simulink model "bldc_sixstep_f28069mLaunchPad"  (R2023b)
settings: Solver=FixedStepAuto  StartTime=0.0  StopTime=1.6  RelTol=1e-3  EnableMultiTasking=on
values from neighbouring files (symbols this model uses):
  bldc = mcb_SetPMSMMotorParameters('Teknic2310P')    [bldc_sixstep_f28069mLaunchPad_data.m]    (also in projectData.mat = )
  inverter = mcb_SetInverterParameters('BoostXL-DRV8305')    [bldc_sixstep_f28069mLaunchPad_data.m]    (also in projectData.mat = )
  PI_params = mcb_SetControllerParameters(bldc,inverter,PU_System,T_pwm,2*Ts,Ts_speed)    [bldc_sixstep_f28069mLaunchPad_data.m]    (also in projectData.mat = )
  PWM_frequency = 20e3    (= 20000)    [bldc_sixstep_f28069mLaunchPad_data.m]    (also in projectData.mat)
  target = mcb_SetProcessorDetails('F28069M',PWM_frequency)    [bldc_sixstep_f28069mLaunchPad_data.m]    (also in projectData.mat = )
  Ts = T_pwm    (= 5e-05)    [bldc_sixstep_f28069mLaunchPad_data.m]    (also in projectData.mat)
  Ts_motor_simscape = T_pwm/100    (= 5e-07)    [bldc_sixstep_f28069mLaunchPad_data.m]    (also in projectData.mat)
  Ts_simulink = T_pwm/2    (= 2.5e-05)    [bldc_sixstep_f28069mLaunchPad_data.m]    (also in projectData.mat)
  Ts_speed = 10*Ts    (= 0.0005)    [bldc_sixstep_f28069mLaunchPad_data.m]    (also in projectData.mat)
libraries: nesl_utility x14, fl_lib x9, mcbcontrolslib x7, simulink x6, pil_lib x6, ee_lib x5, slpidlib x4, mcbpositiondecoderlib x4
(part 1 of 3)
settings Model: ExtModeTrigDuration=8  Creator=Tefilus  LastModifiedBy=Tefilus
settings SolverCC: AutoInsertRateTranBlk=on
settings OptimizationCC: DefaultParameterBehavior=Inlined  DefaultUnderspecifiedDataType=single  EnhancedBackFolding=on  PassReuseOutputArgsAs=Individual arguments  MaxStackSize=1024  OptimizeBlockOrder=speed  DifferentSizesBufferReuse=on  OptimizationCustomize=off  DenormalBehavior=FlushToZero  EfficientTunableParamExpr=on
settings DebuggingCC: ParameterPrecisionLossMsg=none  ParameterTunabilityLossMsg=error
settings HardwareCC: ProdBitPerChar=16  ProdBitPerInt=16  ProdBitPerPointer=32  ProdBitPerSizeT=32  ProdBitPerPtrDiffT=32  ProdLargestAtomicInteger=Integer  ProdLargestAtomicFloat=None  ProdWordSize=16  ProdLongLongMode=on  ProdHWDeviceType=Texas Instruments->C2000  HardwareBoardFeatureSet=SoCBlockset
settings ModelReferenceCC: ModelReferenceNumInstancesAllowed=Single
settings SFSimCC: MATLABDynamicMemAlloc=off
settings RTWCC: Description=Embedded Coder  SystemTargetFile=ert.tlc  HardwareBoard=TI Piccolo F28069M LaunchPad  TemplateMakefile=ert_default_tmf  Toolchain=Texas Instruments Code Composer Studio (C2000)  PortableWordSizes=on  CreateSILPILBlock=PIL  CodeExecutionProfiling=on  CodeProfilingInstrumentation=coarse
settings CodeAppCC: ForceParamTrailComments=on  IgnoreCustomStorageClasses=off  OperatorAnnotations=on  SimulinkDataObjDesc=on  SFDataObjDesc=on  InsertBlockDesc=on
settings ERTTargetCC: CodeReplacementLibrary=TI C28x  ExtModeTransport=4  ExtModeStaticAlloc=on  ExtModeAutomaticAllocSize=off  ExtModeStaticAllocSize=2000  ExtModeMexFile=ext_xcp  ExtModeIntrfLevel=Level2 - Open  InlinedParameterPlacement=NonHierarchical

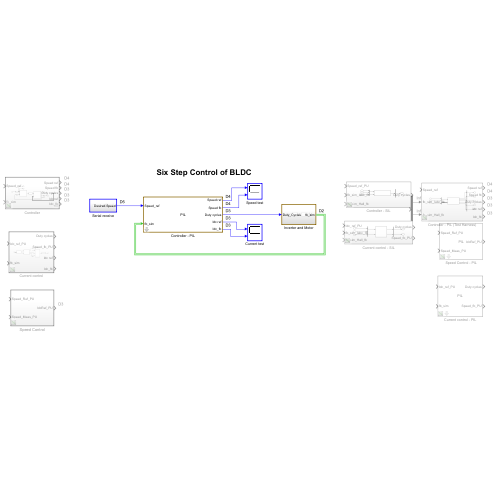
[thumbnail: Simulink's stored preview of the top-level diagram]
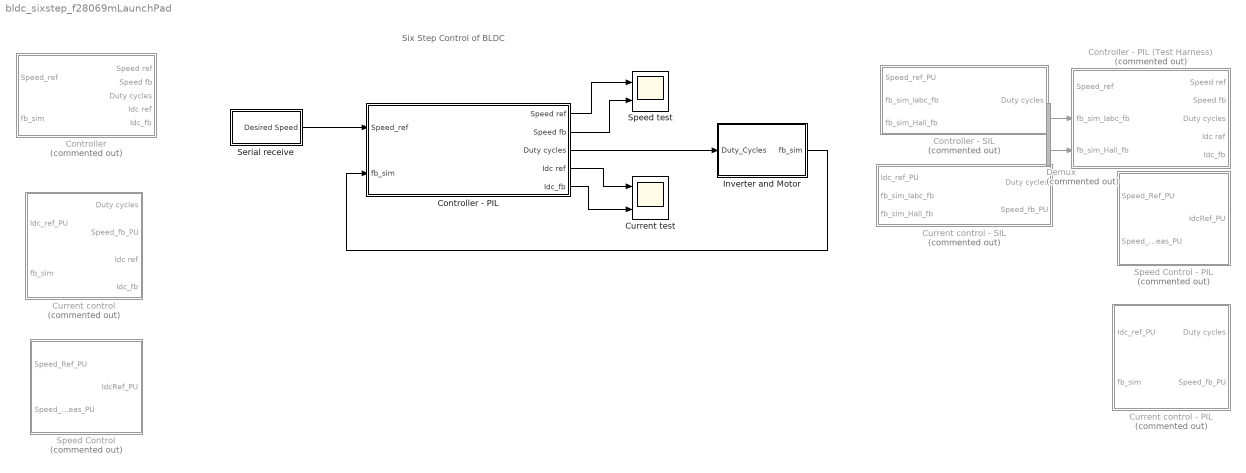
== system bldc_sixstep_f28069mLaunchPad ==
  note: Six Step Control of BLDC
  Controller : Subsystem  Commented=on  TreatAsAtomicUnit=on
  Controller - PIL : Subsystem  DialogController=pil_create_dialog  LoadFcn=|
      | try
      |    if ~strcmp(rtw.pil.getPILVersion, '23.2 (R2023b)_15')
      |       set_param(gcb, 'DialogController', '');
      |       set_param(gcb, 'DialogControllerArgs', '');
      |    end
      | catch e
      |       set_param(gcb, 'DialogController', '');
      |       set_param(gcb, 'DialogControllerArgs', '');
      | end
      mask help: PIL:pil:XILBlockMaskDesc
      mask Display: disp('PIL');
  Controller - PIL (Test Harness) : Subsystem  Commented=on
  Controller - SIL : Subsystem  Commented=on
  Current control : Subsystem  Commented=on  TreatAsAtomicUnit=on  SystemSampleTime=Ts
  Current control - PIL : Subsystem  Commented=on  DialogController=pil_create_dialog  LoadFcn=|
      | try
      |    if ~strcmp(rtw.pil.getPILVersion, '23.2 (R2023b)_15')
      |       set_param(gcb, 'DialogController', '');
      |       set_param(gcb, 'DialogControllerArgs', '');
      |    end
      | catch e
      |       set_param(gcb, 'DialogController', '');
      |       set_param(gcb, 'DialogControllerArgs', '');
      | end
      mask help: PIL:pil:XILBlockMaskDesc
      mask Display: disp('PIL');
  Current control - SIL : Subsystem  Commented=on
  Current test : Scope  NumInputPorts=2
  Demux : Demux  Commented=on  Outputs=2
  Inverter and Motor : Subsystem
  Serial receive : Subsystem  TreatAsAtomicUnit=on  SystemSampleTime=0.1
  Speed Control : Subsystem  Commented=on  TreatAsAtomicUnit=on  SystemSampleTime=Ts_speed
  Speed Control - PIL : Subsystem  Commented=on  DialogController=pil_create_dialog  LoadFcn=|
      | try
      |    if ~strcmp(rtw.pil.getPILVersion, '23.2 (R2023b)_15')
      |       set_param(gcb, 'DialogController', '');
      |       set_param(gcb, 'DialogControllerArgs', '');
      |    end
      | catch e
      |       set_param(gcb, 'DialogController', '');
      |       set_param(gcb, 'DialogControllerArgs', '');
      | end
      mask help: PIL:pil:XILBlockMaskDesc
      mask Display: disp('PIL');
  Speed test : Scope  NumInputPorts=2
  wires:
  Demux/1 -> Controller - PIL (Test Harness)/2(fb_sim_Iabc_fb)
  Demux/2 -> Controller - PIL (Test Harness)/3(fb_sim_Hall_fb)
  Controller - PIL/1(Speed ref) -> Speed test/1
  Controller - PIL/2(Speed fb) -> Speed test/2
  Controller - PIL/4(Idc ref) -> Current test/1
  Controller - PIL/5(Idc_fb) -> Current test/2
  Serial receive/1(Desired Speed) -> Controller - PIL/1(Speed_ref)
  Controller - PIL/3(Duty cycles) -> Inverter and Motor/1(Duty_Cycles)
  Inverter and Motor/1(fb_sim) -> Controller - PIL/2(fb_sim)

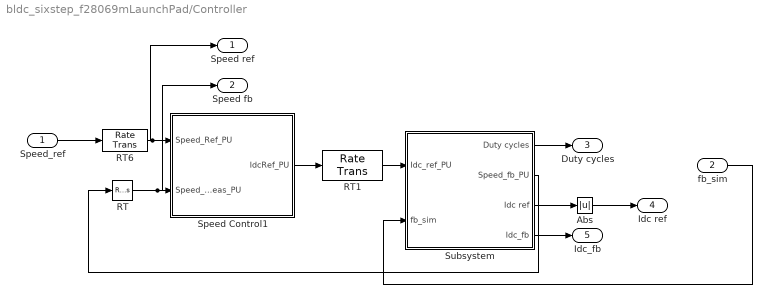
== system bldc_sixstep_f28069mLaunchPad/Controller ==
  Speed_ref : Inport
  fb_sim : Inport  Port=2
  Abs : Abs  SaturateOnIntegerOverflow=off
  RT : RateTransition  OutPortSampleTime=0.0005
  RT1 : RateTransition  Deterministic=off
  RT6 : RateTransition  Deterministic=off
  Speed Control1 : Subsystem  TreatAsAtomicUnit=on  SystemSampleTime=Ts_speed
  Subsystem : Subsystem  TreatAsAtomicUnit=on  SystemSampleTime=Ts
  Speed ref : Outport
  Speed fb : Outport  Port=2
  Duty cycles : Outport  Port=3
  Idc ref : Outport  Port=4
  Idc_fb : Outport  Port=5
  wires:
  Subsystem/2(Speed_fb_PU) -> RT/1
  RT6/1 -> Speed ref/1, Speed Control1/1(Speed_Ref_PU)
  Subsystem/1(Duty cycles) -> Duty cycles/1
  RT/1 -> Speed fb/1, Speed Control1/2(Speed_Meas_PU)
  Speed Control1/1(IdcRef_PU) -> RT1/1
  RT1/1 -> Subsystem/1(Idc_ref_PU)
  Speed_ref/1 -> RT6/1
  fb_sim/1 -> Subsystem/2(fb_sim)
  Subsystem/3(Idc ref) -> Abs/1
  Subsystem/4(Idc_fb) -> Idc_fb/1
  Abs/1 -> Idc ref/1

== system bldc_sixstep_f28069mLaunchPad/Controller - PIL ==
  Speed_ref : Inport
  fb_sim : Inport  Port=2
  Controller_sfcn : pil_lib/PIL Block  SimulationMode=PIL  IsTopModelPIL=off  CodeDir=Controller_ert_rtw  AnchorDir=E:\GiaotrinhDH\DATN\exampleSIL_PIL_MIL_HIL\SixStep_QEP  ConfigName=Texas Instruments C2000 Base  XrelIsTopModelCode=on  XrelIsReusable=off  XrelDWorkNames={}  XrelDWorkTypes={}  XrelModelArgVals={}  XrelOrderedParamNames={}
  __InputSSForSFun__ : Subsystem
  __OutputSSForSFun__ : Subsystem
  Speed ref : Outport
  Speed fb : Outport  Port=2
  Duty cycles : Outport  Port=3
  Idc ref : Outport  Port=4
  Idc_fb : Outport  Port=5
  wires:
  Speed_ref/1 -> __InputSSForSFun__/1(Speed_ref)
  fb_sim/1 -> __InputSSForSFun__/2(fb_sim)
  __InputSSForSFun__/1(__UniqueOutportName__1__) -> Controller_sfcn/1
  __InputSSForSFun__/2(__UniqueOutportName__2__) -> Controller_sfcn/2
  __InputSSForSFun__/3(__UniqueOutportName__3__) -> Controller_sfcn/3
  Controller_sfcn/1 -> __OutputSSForSFun__/1(__UniqueInportName__1__)
  Controller_sfcn/2 -> __OutputSSForSFun__/2(__UniqueInportName__2__)
  Controller_sfcn/3 -> __OutputSSForSFun__/3(__UniqueInportName__3__)
  Controller_sfcn/4 -> __OutputSSForSFun__/4(__UniqueInportName__4__)
  Controller_sfcn/5 -> __OutputSSForSFun__/5(__UniqueInportName__5__)
  __OutputSSForSFun__/1(Speed ref) -> Speed ref/1
  __OutputSSForSFun__/2(Speed fb) -> Speed fb/1
  __OutputSSForSFun__/3(Duty cycles) -> Duty cycles/1
  __OutputSSForSFun__/4(Idc ref) -> Idc ref/1
  __OutputSSForSFun__/5(Idc_fb) -> Idc_fb/1

== system bldc_sixstep_f28069mLaunchPad/Controller - PIL (Test Harness) ==
  Speed_ref : Inport  OutDataTypeStr=single  PortDimensions=[1]  SampleTime=0.1
  fb_sim_Iabc_fb : Inport  Port=2  OutDataTypeStr=uint16  PortDimensions=[3]  SampleTime=2.5e-05
  fb_sim_Hall_fb : Inport  Port=3  OutDataTypeStr=uint32  PortDimensions=[3]  SampleTime=5e-05
  Controller1 : Subsystem  Tag=__SL_testing_harness_stub_  DialogController=pil_create_dialog  LoadFcn=|
      | try
      |    if ~strcmp(rtw.pil.getPILVersion, '23.2 (R2023b)_15')
      |       set_param(gcb, 'DialogController', '');
      |       set_param(gcb, 'DialogControllerArgs', '');
      |    end
      | catch e
      |       set_param(gcb, 'DialogController', '');
      |       set_param(gcb, 'DialogControllerArgs', '');
      | end
      mask help: PIL:pil:XILBlockMaskDesc
      mask Display: disp('PIL');
  Input Conversion Subsystem : Subsystem  Tag=__SLT_ICS__  Description=|
      | Signal spec.
      | and routing
      settings: AttributesFormatString=%<Description>
  Output Conversion Subsystem : Subsystem  Tag=__SLT_OCS__  Description=|
      | Signal spec.
      | and routing
      settings: AttributesFormatString=%<Description>
  Speed ref : Outport
  Speed fb : Outport  Port=2
  Duty cycles : Outport  Port=3
  Idc ref : Outport  Port=4
  Idc_fb : Outport  Port=5
  wires:
  Controller1/2(Speed fb) -> Output Conversion Subsystem/2(Inport_2)
  Output Conversion Subsystem/2(Outport_2) -> Speed fb/1
  Output Conversion Subsystem/4(Outport_4) -> Idc ref/1
  Input Conversion Subsystem/1(Outport_1) -> Controller1/1(Speed_ref)
  Output Conversion Subsystem/3(Outport_3) -> Duty cycles/1
  Output Conversion Subsystem/5(Outport_5) -> Idc_fb/1
  fb_sim_Iabc_fb/1 -> Input Conversion Subsystem/2(Inport_2)
  Controller1/4(Idc ref) -> Output Conversion Subsystem/4(Inport_4)
  Controller1/3(Duty cycles) -> Output Conversion Subsystem/3(Inport_3)
  fb_sim_Hall_fb/1 -> Input Conversion Subsystem/3(Inport_3)
  Speed_ref/1 -> Input Conversion Subsystem/1(Inport_1)
  Output Conversion Subsystem/1(Outport_1) -> Speed ref/1
  Input Conversion Subsystem/2(Outport_2) -> Controller1/2(fb_sim)
  Controller1/1(Speed ref) -> Output Conversion Subsystem/1(Inport_1)
  Controller1/5(Idc_fb) -> Output Conversion Subsystem/5(Inport_5)

== system bldc_sixstep_f28069mLaunchPad/Controller - SIL ==
  Speed_ref_PU : Inport  OutDataTypeStr=single  PortDimensions=[1]  SampleTime=0.1
  fb_sim_Iabc_fb : Inport  Port=2  OutDataTypeStr=uint16  PortDimensions=[3]  SampleTime=2.5e-05
  fb_sim_Hall_fb : Inport  Port=3  OutDataTypeStr=uint32  PortDimensions=[3]  SampleTime=2.5e-05
  Input Conversion Subsystem : Subsystem  Tag=__SLT_ICS__  Description=|
      | Signal spec.
      | and routing
      settings: AttributesFormatString=%<Description>
  Output Conversion Subsystem : Subsystem  Tag=__SLT_OCS__  Description=|
      | Signal spec.
      | and routing
      settings: AttributesFormatString=%<Description>
  Subsystem : Subsystem  Tag=__SL_testing_harness_stub_  DialogController=pil_create_dialog  LoadFcn=|
      | try
      |    if ~strcmp(rtw.pil.getPILVersion, '23.2 (R2023b)_15')
      |       set_param(gcb, 'DialogController', '');
      |       set_param(gcb, 'DialogControllerArgs', '');
      |    end
      | catch e
      |       set_param(gcb, 'DialogController', '');
      |       set_param(gcb, 'DialogControllerArgs', '');
      | end
      mask help: PIL:pil:XILBlockMaskDesc
      mask Display: disp('SIL');
  Duty cycles : Outport
  wires:
  Speed_ref_PU/1 -> Input Conversion Subsystem/1(Inport_1)
  Input Conversion Subsystem/2(Outport_2) -> Subsystem/2(fb_sim)
  fb_sim_Hall_fb/1 -> Input Conversion Subsystem/3(Inport_3)
  fb_sim_Iabc_fb/1 -> Input Conversion Subsystem/2(Inport_2)
  Subsystem/1(Duty cycles) -> Output Conversion Subsystem/1(Inport_1)
  Output Conversion Subsystem/1(Outport_1) -> Duty cycles/1
  Input Conversion Subsystem/1(Outport_1) -> Subsystem/1(Speed_ref_PU)

== system bldc_sixstep_f28069mLaunchPad/Current control ==
  Idc_ref_PU : Inport
  fb_sim : Inport  Port=2
  Control_System : Subsystem
  Input scaling : Subsystem
  Inverter : Subsystem
  Sensor Driver Block : Subsystem
  Duty cycles : Outport
  Speed_fb_PU : Outport  Port=2
  Idc ref : Outport  Port=3
  Idc_fb : Outport  Port=4
  wires:
  fb_sim/1 -> Sensor Driver Block/1(fb_sim)
  Control_System/1(Duty) -> Inverter/1(Inverter Signals)
  Inverter/1(Duty) -> Duty cycles/1
  Idc_ref_PU/1 -> Idc ref/1, Control_System/1(Idc_ref_PU)
  Sensor Driver Block/1(Iabc_Meas_ADC) -> Input scaling/1(Iabc_meas_ADC)
  Sensor Driver Block/2(Hall_Meas) -> Input scaling/2(Hall_Meas)
  Input scaling/2(HallState) -> Control_System/2(Hallstate)
  Input scaling/3(Idc_meas_PU) -> Idc_fb/1, Control_System/3(Idc_fb_PU)
  Input scaling/1(speed_PU) -> Speed_fb_PU/1

== system bldc_sixstep_f28069mLaunchPad/Current control - PIL ==
  Idc_ref_PU : Inport
  fb_sim : Inport  Port=2
  Current control_sfcn : pil_lib/PIL Block  SimulationMode=PIL  IsTopModelPIL=off  CodeDir=Current_ert_rtw  AnchorDir=E:\GiaotrinhDH\DATN\exampleSIL_PIL_MIL_HIL\SixStep_QEP  ConfigName=Texas Instruments C2000 Base  XrelIsTopModelCode=on  XrelIsReusable=off  XrelDWorkNames={}  XrelDWorkTypes={}  XrelModelArgVals={}  XrelOrderedParamNames={}
  Scope : Scope  NumInputPorts=2
  __InputSSForSFun__ : Subsystem
  __OutputSSForSFun__ : Subsystem
  Duty cycles : Outport
  Speed_fb_PU : Outport  Port=2
  wires:
  Idc_ref_PU/1 -> __InputSSForSFun__/1(Idc_ref_PU)
  fb_sim/1 -> __InputSSForSFun__/2(fb_sim)
  __InputSSForSFun__/1(__UniqueOutportName__1__) -> Scope/1, Current control_sfcn/1
  __InputSSForSFun__/2(__UniqueOutportName__2__) -> Scope/2, Current control_sfcn/2
  __InputSSForSFun__/3(__UniqueOutportName__3__) -> Current control_sfcn/3
  Current control_sfcn/1 -> __OutputSSForSFun__/1(__UniqueInportName__1__)
  Current control_sfcn/2 -> __OutputSSForSFun__/2(__UniqueInportName__2__)
  __OutputSSForSFun__/1(Duty cycles) -> Duty cycles/1
  __OutputSSForSFun__/2(Speed_fb_PU) -> Speed_fb_PU/1

== system bldc_sixstep_f28069mLaunchPad/Current control - SIL ==
  Idc_ref_PU : Inport  OutDataTypeStr=single  PortDimensions=[1]  SampleTime=5e-05
  fb_sim_Iabc_fb : Inport  Port=2  OutDataTypeStr=uint16  PortDimensions=[3]  SampleTime=2.5e-05
  fb_sim_Hall_fb : Inport  Port=3  OutDataTypeStr=uint32  PortDimensions=[3]  SampleTime=2.5e-05
  Current control - SIL : Subsystem  Tag=__SL_testing_harness_stub_  DialogController=pil_create_dialog  LoadFcn=|
      | try
      |    if ~strcmp(rtw.pil.getPILVersion, '23.2 (R2023b)_15')
      |       set_param(gcb, 'DialogController', '');
      |       set_param(gcb, 'DialogControllerArgs', '');
      |    end
      | catch e
      |       set_param(gcb, 'DialogController', '');
      |       set_param(gcb, 'DialogControllerArgs', '');
      | end
      mask help: PIL:pil:XILBlockMaskDesc
      mask Display: disp('SIL');
  Input Conversion Subsystem : Subsystem  Tag=__SLT_ICS__  Description=|
      | Signal spec.
      | and routing
      settings: AttributesFormatString=%<Description>
  Output Conversion Subsystem : Subsystem  Tag=__SLT_OCS__  Description=|
      | Signal spec.
      | and routing
      settings: AttributesFormatString=%<Description>
  Duty cycles : Outport
  Speed_fb_PU : Outport  Port=2
  wires:
  Current control - SIL/1(Duty cycles) -> Output Conversion Subsystem/1(Inport_1)
  Output Conversion Subsystem/2(Outport_2) -> Speed_fb_PU/1
  Input Conversion Subsystem/2(Outport_2) -> Current control - SIL/2(fb_sim)
  fb_sim_Iabc_fb/1 -> Input Conversion Subsystem/2(Inport_2)
  Input Conversion Subsystem/1(Outport_1) -> Current control - SIL/1(Idc_ref_PU)
  Output Conversion Subsystem/1(Outport_1) -> Duty cycles/1
  fb_sim_Hall_fb/1 -> Input Conversion Subsystem/3(Inport_3)
  Current control - SIL/2(Speed_fb_PU) -> Output Conversion Subsystem/2(Inport_2)
  Idc_ref_PU/1 -> Input Conversion Subsystem/1(Inport_1)

== system bldc_sixstep_f28069mLaunchPad/Inverter and Motor ==
  Duty_Cycles : Inport
  Bus Creator : BusCreator  Inputs=2
  Inverter and Motor : Subsystem  VariantControl=get_param([bdroot '/Plant'],'Value')=='0'
  Load_Profile (Torque) : Subsystem
  RT2 : RateTransition  Deterministic=off  OutPortSampleTime=Ts_simulink
  RT3 : RateTransition  Deterministic=off  OutPortSampleTime=Ts_simulink
  Sensor_Measurements : Subsystem
  fb_sim : Outport
  wires:
  RT3/1 -> Sensor_Measurements/1(Iabc meas)
  Sensor_Measurements/2(HallState) -> Bus Creator/2  "Hall_fb"
  Inverter and Motor/2(Hall) -> RT2/1
  Sensor_Measurements/1(Iabc meas ADC) -> Bus Creator/1  "Iabc_fb"
  RT2/1 -> Sensor_Measurements/2(Hall)
  Load_Profile (Torque)/1(Load_Trq) -> Inverter and Motor/2(Load)
  Inverter and Motor/1(Iabc) -> RT3/1
  Duty_Cycles/1 -> Inverter and Motor/1(Duty_Cycles)
  Bus Creator/1 -> fb_sim/1

== system bldc_sixstep_f28069mLaunchPad/Serial receive ==
  Data Type Conversion1 : DataTypeConversion  OutDataTypeStr=dataType  RndMeth=Simplest  SaturateOnIntegerOverflow=off
  Data Type Conversion3 : DataTypeConversion  OutDataTypeStr=boolean  RndMeth=Simplest  SaturateOnIntegerOverflow=off
  Data conditioning : Subsystem
  Demux1 : Demux  Outputs=2
  SCI_Rx : Subsystem
  Terminator : Terminator
  Desired Speed : Outport  VectorParamsAs1DForOutWhenUnconnected=off
  wires:
  SCI_Rx/1(Data) -> Data conditioning/1(Rx_In)
  Demux1/1 -> Data Type Conversion1/1
  Demux1/2 -> Data Type Conversion3/1
  Data Type Conversion1/1 -> Desired Speed/1
  Data conditioning/1(Rx_Out) -> Demux1/1
  Data Type Conversion3/1 -> Terminator/1

== system bldc_sixstep_f28069mLaunchPad/Speed Control ==
  Speed_Ref_PU : Inport
  Speed_Meas_PU : Inport  Port=2
  PI_Controller_Speed : Subsystem
  Scope : Scope  NumInputPorts=2
  Speed_Ref_Selector : Subsystem
  IdcRef_PU : Outport  VectorParamsAs1DForOutWhenUnconnected=off
  wires:
  PI_Controller_Speed/1(Idc_ref) -> IdcRef_PU/1
  Speed_Meas_PU/1 -> Scope/2, PI_Controller_Speed/2(N_fb), Speed_Ref_Selector/2(Speed_Ref_Open)  "Speed_fb"
  Speed_Ref_PU/1 -> Scope/1, Speed_Ref_Selector/1(Speed_Ref_In)  "SpeedRef"
  Speed_Ref_Selector/1(Speed_Ref_PU) -> PI_Controller_Speed/1(N_ref)  "Speed_Ref"

== system bldc_sixstep_f28069mLaunchPad/Speed Control - PIL ==
  Speed_Ref_PU : Inport
  Speed_Meas_PU : Inport  Port=2
  Speed Control_sfcn : pil_lib/PIL Block  SimulationMode=PIL  IsTopModelPIL=off  CodeDir=Speed_ert_rtw  AnchorDir=E:\GiaotrinhDH\DATN\exampleSIL_PIL_MIL_HIL\SixStep_QEP  ConfigName=Texas Instruments C2000 Base  XrelIsTopModelCode=on  XrelIsReusable=off  XrelDWorkNames={}  XrelDWorkTypes={}  XrelModelArgVals={}  XrelOrderedParamNames={}
  __InputSSForSFun__ : Subsystem
  __OutputSSForSFun__ : Subsystem
  IdcRef_PU : Outport  VectorParamsAs1DForOutWhenUnconnected=off
  wires:
  Speed_Ref_PU/1 -> __InputSSForSFun__/1(Speed_Ref_PU)
  Speed_Meas_PU/1 -> __InputSSForSFun__/2(Speed_Meas_PU)
  __InputSSForSFun__/1(__UniqueOutportName__1__) -> Speed Control_sfcn/1
  __InputSSForSFun__/2(__UniqueOutportName__2__) -> Speed Control_sfcn/2
  Speed Control_sfcn/1 -> __OutputSSForSFun__/1(__UniqueInportName__1__)
  __OutputSSForSFun__/1(IdcRef_PU) -> IdcRef_PU/1

== system bldc_sixstep_f28069mLaunchPad/Controller/Speed Control1 ==
  Speed_Ref_PU : Inport
  Speed_Meas_PU : Inport  Port=2
  PI_Controller_Speed : Subsystem
  Scope : Scope  NumInputPorts=2
  Speed_Ref_Selector : Subsystem
  IdcRef_PU : Outport  VectorParamsAs1DForOutWhenUnconnected=off
  wires:
  PI_Controller_Speed/1(Idc_ref) -> IdcRef_PU/1
  Speed_Meas_PU/1 -> Scope/2, PI_Controller_Speed/2(N_fb), Speed_Ref_Selector/2(Speed_Ref_Open)  "Speed_fb"
  Speed_Ref_PU/1 -> Scope/1, Speed_Ref_Selector/1(Speed_Ref_In)  "SpeedRef"
  Speed_Ref_Selector/1(Speed_Ref_PU) -> PI_Controller_Speed/1(N_ref)  "Speed_Ref"

== system bldc_sixstep_f28069mLaunchPad/Controller/Subsystem ==
  Idc_ref_PU : Inport
  fb_sim : Inport  Port=2
  Control_System : Subsystem
  Input scaling : Subsystem
  Inverter : Subsystem
  Sensor Driver Block : Subsystem
  Duty cycles : Outport
  Speed_fb_PU : Outport  Port=2
  Idc ref : Outport  Port=3
  Idc_fb : Outport  Port=4
  wires:
  fb_sim/1 -> Sensor Driver Block/1(fb_sim)
  Control_System/1(Duty) -> Inverter/1(Inverter Signals)
  Inverter/1(Duty) -> Duty cycles/1
  Idc_ref_PU/1 -> Idc ref/1, Control_System/1(Idc_ref_PU)
  Sensor Driver Block/1(Iabc_Meas_ADC) -> Input scaling/1(Iabc_meas_ADC)
  Sensor Driver Block/2(Hall_Meas) -> Input scaling/2(Hall_Meas)
  Input scaling/2(HallState) -> Control_System/2(Hallstate)
  Input scaling/3(Idc_meas_PU) -> Idc_fb/1, Control_System/3(Idc_fb_PU)
  Input scaling/1(speed_PU) -> Speed_fb_PU/1

== system bldc_sixstep_f28069mLaunchPad/Controller - PIL/__InputSSForSFun__ ==
  Speed_ref : Inport
  fb_sim : Inport  Port=2
  temporaryBusSelectName_1 : BusSelector  OutputSignals=Iabc_fb,Hall_fb
  __UniqueOutportName__1__ : Outport
  __UniqueOutportName__2__ : Outport  Port=2
  __UniqueOutportName__3__ : Outport  Port=3
  wires:
  fb_sim/1 -> temporaryBusSelectName_1/1
  Speed_ref/1 -> __UniqueOutportName__1__/1
  temporaryBusSelectName_1/1 -> __UniqueOutportName__2__/1  "<Iabc_fb>"
  temporaryBusSelectName_1/2 -> __UniqueOutportName__3__/1  "<Hall_fb>"

== system bldc_sixstep_f28069mLaunchPad/Controller - PIL/__OutputSSForSFun__ ==
  __UniqueInportName__1__ : Inport
  __UniqueInportName__2__ : Inport  Port=2
  __UniqueInportName__3__ : Inport  Port=3
  __UniqueInportName__4__ : Inport  Port=4
  __UniqueInportName__5__ : Inport  Port=5
  Speed ref : Outport
  Speed fb : Outport  Port=2
  Duty cycles : Outport  Port=3
  Idc ref : Outport  Port=4
  Idc_fb : Outport  Port=5
  wires:
  __UniqueInportName__1__/1 -> Speed ref/1
  __UniqueInportName__2__/1 -> Speed fb/1
  __UniqueInportName__3__/1 -> Duty cycles/1
  __UniqueInportName__4__/1 -> Idc ref/1
  __UniqueInportName__5__/1 -> Idc_fb/1  "IDC"

== system bldc_sixstep_f28069mLaunchPad/Controller - PIL (Test Harness)/Controller1 ==
  Speed_ref : Inport
  fb_sim : Inport  Port=2
  Controller_sfcn : pil_lib/PIL Block  SimulationMode=PIL  IsTopModelPIL=off  CodeDir=Controller_ert_rtw  AnchorDir=E:\GiaotrinhDH\DATN\exampleSIL_PIL_MIL_HIL\SixStep_QEP  ConfigName=Texas Instruments C2000 Base  XrelIsTopModelCode=on  XrelIsReusable=off  XrelDWorkNames={}  XrelDWorkTypes={}  XrelModelArgVals={}  XrelOrderedParamNames={}
  __InputSSForSFun__ : Subsystem
  __OutputSSForSFun__ : Subsystem
  Speed ref : Outport
  Speed fb : Outport  Port=2
  Duty cycles : Outport  Port=3
  Idc ref : Outport  Port=4
  Idc_fb : Outport  Port=5
  wires:
  __OutputSSForSFun__/5(Idc_fb) -> Idc_fb/1
  __OutputSSForSFun__/4(Idc ref) -> Idc ref/1
  __OutputSSForSFun__/3(Duty cycles) -> Duty cycles/1
  __OutputSSForSFun__/2(Speed fb) -> Speed fb/1
  __OutputSSForSFun__/1(Speed ref) -> Speed ref/1
  Controller_sfcn/5 -> __OutputSSForSFun__/5(__UniqueInportName__5__)
  Controller_sfcn/4 -> __OutputSSForSFun__/4(__UniqueInportName__4__)
  Controller_sfcn/3 -> __OutputSSForSFun__/3(__UniqueInportName__3__)
  Controller_sfcn/2 -> __OutputSSForSFun__/2(__UniqueInportName__2__)
  Controller_sfcn/1 -> __OutputSSForSFun__/1(__UniqueInportName__1__)
  __InputSSForSFun__/3(__UniqueOutportName__3__) -> Controller_sfcn/3
  __InputSSForSFun__/2(__UniqueOutportName__2__) -> Controller_sfcn/2
  __InputSSForSFun__/1(__UniqueOutportName__1__) -> Controller_sfcn/1
  fb_sim/1 -> __InputSSForSFun__/2(fb_sim)
  Speed_ref/1 -> __InputSSForSFun__/1(Speed_ref)

== system bldc_sixstep_f28069mLaunchPad/Controller - PIL (Test Harness)/Input Conversion Subsystem ==
  note: This subsystem has been inserted by Simulink to adapt the output of the source blocks to the interface required by the harnessed component.
      |  Modifying the contents of this subsystem may result in compilation and simulation failure.
  Inport_1 : Inport
  Inport_2 : Inport  Port=2
  Inport_3 : Inport  Port=3
  BusCreator_1 : BusCreator  Inputs=2
  SigSpec_1 : SignalSpecification  OutDataTypeStr=single  Dimensions=[1]  SampleTime=0.1
  SigSpec_2 : SignalSpecification  OutDataTypeStr=uint16  Dimensions=[3]  SampleTime=2.5e-05
  SigSpec_3 : SignalSpecification  OutDataTypeStr=uint32  Dimensions=[3]  SampleTime=5e-05
  Outport_1 : Outport
  Outport_2 : Outport  Port=2
  wires:
  SigSpec_1/1 -> Outport_1/1
  Inport_1/1 -> SigSpec_1/1
  BusCreator_1/1 -> Outport_2/1
  SigSpec_2/1 -> BusCreator_1/1
  Inport_2/1 -> SigSpec_2/1  "Iabc_fb"
  SigSpec_3/1 -> BusCreator_1/2
  Inport_3/1 -> SigSpec_3/1  "Hall_fb"

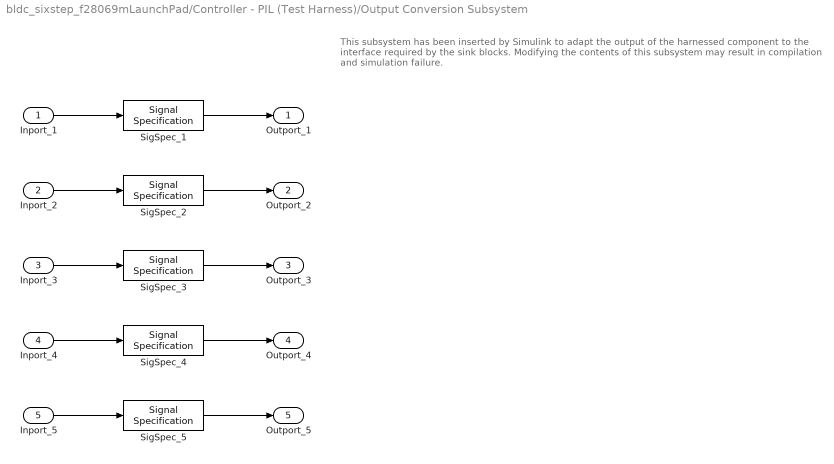
== system bldc_sixstep_f28069mLaunchPad/Controller - PIL (Test Harness)/Output Conversion Subsystem ==
  note: This subsystem has been inserted by Simulink to adapt the output of the harnessed component to the interface required by the sink blocks.
      |  Modifying the contents of this subsystem may result in compilation and simulation failure.
  Inport_1 : Inport
  Inport_2 : Inport  Port=2
  Inport_3 : Inport  Port=3
  Inport_4 : Inport  Port=4
  Inport_5 : Inport  Port=5
  SigSpec_1 : SignalSpecification  OutDataTypeStr=single  Dimensions=[1]  SampleTime=0.0005
  SigSpec_2 : SignalSpecification  OutDataTypeStr=single  Dimensions=[1]  SampleTime=0.0005
  SigSpec_3 : SignalSpecification  OutDataTypeStr=single  Dimensions=[6]  SampleTime=5e-05
  SigSpec_4 : SignalSpecification  OutDataTypeStr=single  Dimensions=[1]  SampleTime=5e-05
  SigSpec_5 : SignalSpecification  OutDataTypeStr=single  Dimensions=[1]  SampleTime=5e-05
  Outport_1 : Outport
  Outport_2 : Outport  Port=2
  Outport_3 : Outport  Port=3
  Outport_4 : Outport  Port=4
  Outport_5 : Outport  Port=5
  wires:
  Inport_1/1 -> SigSpec_1/1
  SigSpec_1/1 -> Outport_1/1
  Inport_2/1 -> SigSpec_2/1
  SigSpec_2/1 -> Outport_2/1
  Inport_3/1 -> SigSpec_3/1
  SigSpec_3/1 -> Outport_3/1
  Inport_4/1 -> SigSpec_4/1
  SigSpec_4/1 -> Outport_4/1
  Inport_5/1 -> SigSpec_5/1
  SigSpec_5/1 -> Outport_5/1

== system bldc_sixstep_f28069mLaunchPad/Controller - SIL/Input Conversion Subsystem ==
  note: This subsystem has been inserted by Simulink to adapt the output of the source blocks to the interface required by the harnessed component.
      |  Modifying the contents of this subsystem may result in compilation and simulation failure.
  Inport_1 : Inport
  Inport_2 : Inport  Port=2
  Inport_3 : Inport  Port=3
  BusCreator_1 : BusCreator  Inputs=2
  SigSpec_1 : SignalSpecification  OutDataTypeStr=single  Dimensions=[1]  SampleTime=0.1
  SigSpec_2 : SignalSpecification  OutDataTypeStr=uint16  Dimensions=[3]  SampleTime=2.5e-05
  SigSpec_3 : SignalSpecification  OutDataTypeStr=uint32  Dimensions=[3]  SampleTime=2.5e-05
  Outport_1 : Outport
  Outport_2 : Outport  Port=2
  wires:
  SigSpec_1/1 -> Outport_1/1
  Inport_1/1 -> SigSpec_1/1
  BusCreator_1/1 -> Outport_2/1
  SigSpec_2/1 -> BusCreator_1/1
  Inport_2/1 -> SigSpec_2/1  "Iabc_fb"
  SigSpec_3/1 -> BusCreator_1/2
  Inport_3/1 -> SigSpec_3/1  "Hall_fb"

== system bldc_sixstep_f28069mLaunchPad/Controller - SIL/Output Conversion Subsystem ==
  note: This subsystem has been inserted by Simulink to adapt the output of the harnessed component to the interface required by the sink blocks.
      |  Modifying the contents of this subsystem may result in compilation and simulation failure.
  Inport_1 : Inport
  SigSpec_1 : SignalSpecification  OutDataTypeStr=single  Dimensions=[6]  SampleTime=5e-05
  Outport_1 : Outport
  wires:
  Inport_1/1 -> SigSpec_1/1
  SigSpec_1/1 -> Outport_1/1

== system bldc_sixstep_f28069mLaunchPad/Controller - SIL/Subsystem ==
  Speed_ref_PU : Inport
  fb_sim : Inport  Port=2
  Subsystem_sfcn : pil_lib/PIL Block  SimulationMode=SIL  IsTopModelPIL=off  CodeDir=Subsystem_ert_rtw  AnchorDir=E:\GiaotrinhDH\DATN\exampleSIL_PIL_MIL_HIL\SixStep_QEP  ConfigName=Software-in-the-Loop (SIL)  XrelIsTopModelCode=on  XrelIsReusable=off  XrelDWorkNames={}  XrelDWorkTypes={}  XrelModelArgVals={}  XrelOrderedParamNames={}
  __InputSSForSFun__ : Subsystem
  __OutputSSForSFun__ : Subsystem
  Duty cycles : Outport
  wires:
  __OutputSSForSFun__/1(Duty cycles) -> Duty cycles/1
  Subsystem_sfcn/1 -> __OutputSSForSFun__/1(__UniqueInportName__1__)
  __InputSSForSFun__/3(__UniqueOutportName__3__) -> Subsystem_sfcn/3
  __InputSSForSFun__/2(__UniqueOutportName__2__) -> Subsystem_sfcn/2
  __InputSSForSFun__/1(__UniqueOutportName__1__) -> Subsystem_sfcn/1
  fb_sim/1 -> __InputSSForSFun__/2(fb_sim)
  Speed_ref_PU/1 -> __InputSSForSFun__/1(Speed_ref_PU)

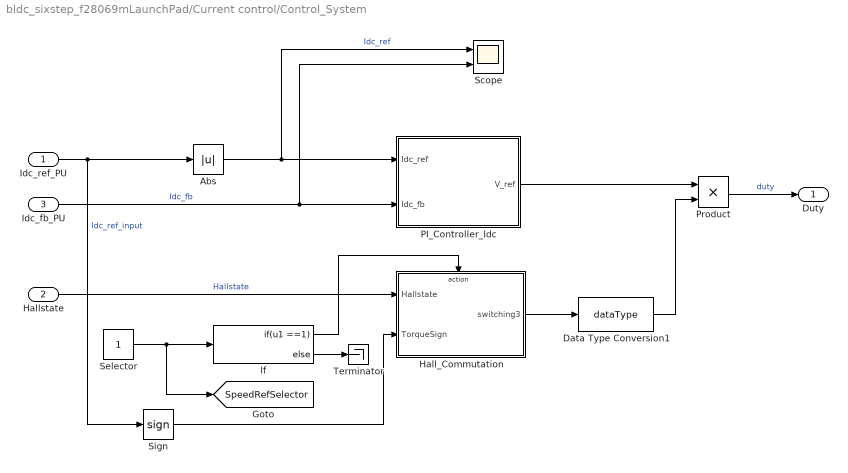
== system bldc_sixstep_f28069mLaunchPad/Current control/Control_System ==
  Idc_ref_PU : Inport
  Hallstate : Inport  Port=2
  Idc_fb_PU : Inport  Port=3
  Abs : Abs  SaturateOnIntegerOverflow=off
  Data Type Conversion1 : DataTypeConversion  OutDataTypeStr=dataType  RndMeth=Simplest  SaturateOnIntegerOverflow=off
  Hall_Commutation : Subsystem
  If : If  IfExpression=u1 ==1
  PI_Controller_Idc : Subsystem
  Product : Product  RndMeth=Simplest  OutDataTypeStr=Inherit: Same as first input
  Scope : Scope  NumInputPorts=2
  Selector : Constant  OutDataTypeStr=uint16  SampleTime=-1
  Sign : Signum
  Terminator : Terminator
  Duty : Outport  VectorParamsAs1DForOutWhenUnconnected=off
  tag scope: SpeedRefSelector=global
  wires:
  Hallstate/1 -> Hall_Commutation/1(Hallstate)  "Hallstate"
  If/1 -> Hall_Commutation/Action
  Idc_fb_PU/1 -> Scope/2, PI_Controller_Idc/2(Idc_fb)  "Idc_fb"
  Abs/1 -> Scope/1, PI_Controller_Idc/1(Idc_ref)  "Idc_ref"
  PI_Controller_Idc/1(V_ref) -> Product/1
  Idc_ref_PU/1 -> Sign/1, Abs/1  "Idc_ref_input"
  Product/1 -> Duty/1  "duty"
  Selector/1 -> If/1, [SpeedRefSelector]
  Sign/1 -> Hall_Commutation/2(TorqueSign)
  Data Type Conversion1/1 -> Product/2
  Hall_Commutation/1(switching3) -> Data Type Conversion1/1
  If/2 -> Terminator/1

== system bldc_sixstep_f28069mLaunchPad/Current control/Input scaling ==
  Iabc_meas_ADC : Inport
  Hall_Meas : Inport  Port=2
  Convert ADC value to PU : Subsystem
  Hall Feedback : Subsystem  TreatAsAtomicUnit=on
  Hall selected : Constant
  If : If  IfExpression=u1 ==1
  Terminator : Terminator
  Terminator1 : Terminator
  speed_PU : Outport  InitialOutput=0  VectorParamsAs1DForOutWhenUnconnected=off
  HallState : Outport  Port=2  InitialOutput=0  VectorParamsAs1DForOutWhenUnconnected=off
  Idc_meas_PU : Outport  Port=3
  wires:
  Hall Feedback/1(HallState) -> HallState/1
  Hall_Meas/1 -> Hall Feedback/1(Hall_Meas)
  If/1 -> Hall Feedback/Action
  Hall selected/1 -> If/1
  Hall Feedback/2(Speed_PU) -> speed_PU/1
  If/2 -> Terminator/1
  Iabc_meas_ADC/1 -> Convert ADC value to PU/1(Iabc_meas_ADC)
  Convert ADC value to PU/1(Idc_meas_PU) -> Idc_meas_PU/1
  Convert ADC value to PU/2(Ia_meas_PU) -> Terminator1/1

== system bldc_sixstep_f28069mLaunchPad/Current control/Inverter ==
  Inverter Signals : Inport
  Constant : Constant
  Data Type Duplicate : DataTypeDuplicate
  Switch : Switch  Threshold=0.5  RndMeth=Simplest  SaturateOnIntegerOverflow=off  InputSameDT=off
  stop : Constant  Value=[0 0 0 0 0 0]  OutDataTypeStr=Inherit: Inherit via back propagation
  Duty : Outport  VectorParamsAs1DForOutWhenUnconnected=off
  wires:
  Constant/1 -> Switch/2
  Switch/1 -> Duty/1
  Inverter Signals/1 -> Switch/1, Data Type Duplicate/1  "PWM Duty Cycles"
  stop/1 -> Switch/3, Data Type Duplicate/2

== system bldc_sixstep_f28069mLaunchPad/Current control/Sensor Driver Block ==
  fb_sim : Inport
  Bus Selector : BusSelector  OutputSignals=Iabc_fb,Hall_fb
  Iabc_Meas_ADC : Outport
  Hall_Meas : Outport  Port=2
  wires:
  Bus Selector/1 -> Iabc_Meas_ADC/1  "<Iabc_fb>"
  fb_sim/1 -> Bus Selector/1
  Bus Selector/2 -> Hall_Meas/1  "<Hall_fb>"

== system bldc_sixstep_f28069mLaunchPad/Current control - PIL/__InputSSForSFun__ ==
  Idc_ref_PU : Inport
  fb_sim : Inport  Port=2
  temporaryBusSelectName_1 : BusSelector  OutputSignals=Iabc_fb,Hall_fb
  __UniqueOutportName__1__ : Outport
  __UniqueOutportName__2__ : Outport  Port=2
  __UniqueOutportName__3__ : Outport  Port=3
  wires:
  fb_sim/1 -> temporaryBusSelectName_1/1
  Idc_ref_PU/1 -> __UniqueOutportName__1__/1
  temporaryBusSelectName_1/1 -> __UniqueOutportName__2__/1  "<Iabc_fb>"
  temporaryBusSelectName_1/2 -> __UniqueOutportName__3__/1  "<Hall_fb>"

== system bldc_sixstep_f28069mLaunchPad/Current control - PIL/__OutputSSForSFun__ ==
  __UniqueInportName__1__ : Inport
  __UniqueInportName__2__ : Inport  Port=2
  Duty cycles : Outport
  Speed_fb_PU : Outport  Port=2
  wires:
  __UniqueInportName__1__/1 -> Duty cycles/1
  __UniqueInportName__2__/1 -> Speed_fb_PU/1

== system bldc_sixstep_f28069mLaunchPad/Current control - SIL/Current control - SIL ==
  Idc_ref_PU : Inport
  fb_sim : Inport  Port=2
  Current control_sfcn : pil_lib/PIL Block  SimulationMode=SIL  IsTopModelPIL=off  CodeDir=Current_ert_rtw  AnchorDir=E:\GiaotrinhDH\DATN\exampleSIL_PIL_MIL_HIL\SixStep_QEP  ConfigName=Software-in-the-Loop (SIL)  XrelIsTopModelCode=on  XrelIsReusable=off  XrelDWorkNames={}  XrelDWorkTypes={}  XrelModelArgVals={}  XrelOrderedParamNames={}
  __InputSSForSFun__ : Subsystem
  __OutputSSForSFun__ : Subsystem
  Duty cycles : Outport
  Speed_fb_PU : Outport  Port=2
  wires:
  __OutputSSForSFun__/2(Speed_fb_PU) -> Speed_fb_PU/1
  __OutputSSForSFun__/1(Duty cycles) -> Duty cycles/1
  Current control_sfcn/2 -> __OutputSSForSFun__/2(__UniqueInportName__2__)
  Current control_sfcn/1 -> __OutputSSForSFun__/1(__UniqueInportName__1__)
  __InputSSForSFun__/3(__UniqueOutportName__3__) -> Current control_sfcn/3
  __InputSSForSFun__/2(__UniqueOutportName__2__) -> Current control_sfcn/2
  __InputSSForSFun__/1(__UniqueOutportName__1__) -> Current control_sfcn/1
  fb_sim/1 -> __InputSSForSFun__/2(fb_sim)
  Idc_ref_PU/1 -> __InputSSForSFun__/1(Idc_ref_PU)

== system bldc_sixstep_f28069mLaunchPad/Current control - SIL/Input Conversion Subsystem ==
  note: This subsystem has been inserted by Simulink to adapt the output of the source blocks to the interface required by the harnessed component.
      |  Modifying the contents of this subsystem may result in compilation and simulation failure.
  Inport_1 : Inport
  Inport_2 : Inport  Port=2
  Inport_3 : Inport  Port=3
  BusCreator_1 : BusCreator  Inputs=2
  SigSpec_1 : SignalSpecification  OutDataTypeStr=single  Dimensions=[1]  SampleTime=5e-05
  SigSpec_2 : SignalSpecification  OutDataTypeStr=uint16  Dimensions=[3]  SampleTime=2.5e-05
  SigSpec_3 : SignalSpecification  OutDataTypeStr=uint32  Dimensions=[3]  SampleTime=2.5e-05
  Outport_1 : Outport
  Outport_2 : Outport  Port=2
  wires:
  SigSpec_1/1 -> Outport_1/1
  Inport_1/1 -> SigSpec_1/1
  BusCreator_1/1 -> Outport_2/1
  SigSpec_2/1 -> BusCreator_1/1
  Inport_2/1 -> SigSpec_2/1  "Iabc_fb"
  SigSpec_3/1 -> BusCreator_1/2
  Inport_3/1 -> SigSpec_3/1  "Hall_fb"

== system bldc_sixstep_f28069mLaunchPad/Current control - SIL/Output Conversion Subsystem ==
  note: This subsystem has been inserted by Simulink to adapt the output of the harnessed component to the interface required by the sink blocks.
      |  Modifying the contents of this subsystem may result in compilation and simulation failure.
  Inport_1 : Inport
  Inport_2 : Inport  Port=2
  SigSpec_1 : SignalSpecification  OutDataTypeStr=single  Dimensions=[6]  SampleTime=5e-05
  SigSpec_2 : SignalSpecification  OutDataTypeStr=single  Dimensions=[1]  SampleTime=5e-05
  Outport_1 : Outport
  Outport_2 : Outport  Port=2
  wires:
  Inport_1/1 -> SigSpec_1/1
  SigSpec_1/1 -> Outport_1/1
  Inport_2/1 -> SigSpec_2/1
  SigSpec_2/1 -> Outport_2/1

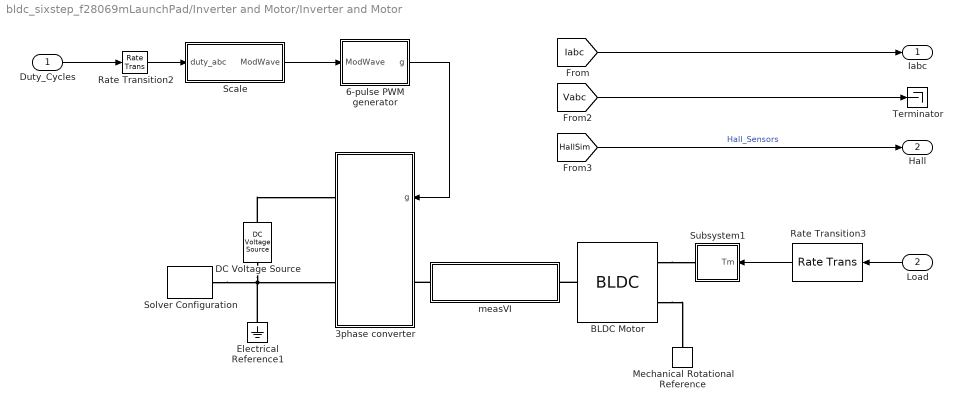
== system bldc_sixstep_f28069mLaunchPad/Inverter and Motor/Inverter and Motor ==
  Duty_Cycles : Inport
  Load : Inport  Port=2
  3phase converter : Subsystem
  6-pulse PWM generator : Subsystem  mask{fs=PWM_frequency}
      mask prompts: fs "Carrier Frequency (Hz)"
  BLDC Motor : ee_lib/Electromechanical/Permanent Magnet/BLDC  port_option=ee.enum.threePhasePort.composite  rotor_param=1  pm_flux_linkage=bldc.FluxPM Wb  theta_constant=pi /(2*bldc.p) rad  emf_max=9.6 V  w_meas=600 rpm  DphiDtheta_tab=[0, -.1528, -.1528, .1528, .1528, 0] Wb/rad  back_emf_tab=[0, -9.6, -9.6, 9.6, 9.6, 0] V  rotor_angle_tab=[0, 7.5, 22.5, 37.5, 52.5, 60] deg  nPolePairs=bldc.p  axes_param=2  winding_type=ee.enum.statorconnection.wye  stator_param=ee.enum.statorparam.LdLqL0  machine_param=ee.enum.dqparameterization.constant  Ld=bldc.Ld H  Lq=bldc.Lq H  idVec=[-200, 0, 200] A  iqVec=[-200, 0, 200] A  LdMatrix=0.00022 * ones(3, 3) H  LqMatrix=0.00022 * ones(3, 3) H  L0=0.00016 H  Ls=0.0002 H  Lm=0 H  Ms=0.00002 H  Rs=bldc.Rs Ohm  zero_sequence=ee.enum.park.zerosequence.exclude  loss_param=ee.enum.ironloss.none  losses_oc=[0, 0, 0] W  losses_sc=[0, 0, 0] W  f_losses=60 Hz  Isc_losses=95 A  J=bldc.J kg*m^2  lam=bldc.B N*m/(rad/s)  i_d_specify=off  i_d_priority=None  i_d=0 A  i_d_nominal_specify=off  i_d_nominal_unit=A  i_d_nominal_value=1  i_q_specify=off  i_q_priority=None  i_q=0 A  i_q_nominal_specify=off  i_q_nominal_unit=A  i_q_nominal_value=1  torque_specify=off  torque_priority=None  torque=0 N*m  torque_nominal_specify=off  torque_nominal_unit=N*m  torque_nominal_value=1  angular_velocity_specify=off  angular_velocity_priority=High  angular_velocity=0 rpm  angular_velocity_nominal_specify=off  angular_velocity_nominal_unit=rpm  angular_velocity_nominal_value=1  angular_position_specify=off  angular_position_priority=High  angular_position=0 deg  angular_position_nominal_specify=off  angular_position_nominal_unit=deg  angular_position_nominal_value=1  alpha=3.93e-3 1/K  alpha_flux=-0.001 1/K  Tmeas=298.15 K  stator_thermal_mass=100 J/K  rotor_thermal_mass=200 J/K  Rm_percent_rotor=90  Rd_percent_rotor=30  temperatureA_specify=off  temperatureA_priority=High  temperatureA=25 degC  temperatureA_nominal_specify=off  temperatureA_nominal_unit=degC  temperatureA_nominal_value=1  temperatureB_specify=off  temperatureB_priority=High  temperatureB=25 degC  temperatureB_nominal_specify=off  temperatureB_nominal_unit=degC  temperatureB_nominal_value=1  temperatureC_specify=off  temperatureC_priority=High  temperatureC=25 degC  temperatureC_nominal_specify=off  temperatureC_nominal_unit=degC  temperatureC_nominal_value=1  temperatureR_specify=off  temperatureR_priority=High  temperatureR=25 degC  temperatureR_nominal_specify=off  temperatureR_nominal_unit=degC  temperatureR_nominal_value=1
      settings: InternalSimscapePortConfiguration="{\"Bottom\":[],\"Left\":[{\"id\":\"N\",\"label\":\"~\",\"type\":\"foundation.electrical.three_phase\"}],\"Right\":[{\"id\":\"R\",\"label\":\"R\",\"type\":\"foundation.mechanical.rotational.rotational\"},{\"id\":\"C\",\"label\":\"C\",\"type\":\"foundation.mechanical.rotational.rotational\"}],\"Top\":[]}"
  DC Voltage Source : fl_lib/Electrical/Electrical Sources/DC Voltage Source  v0=inverter.V_dc V
  Electrical Reference1 : fl_lib/Electrical/Electrical Elements/Electrical Reference
  Mechanical Rotational Reference : fl_lib/Mechanical/Rotational Elements/Mechanical Rotational Reference
  Rate Transition2 : RateTransition  Deterministic=off  OutPortSampleTime=Ts_motor_simscape
  Rate Transition3 : RateTransition  Deterministic=off  OutPortSampleTime=Ts_motor_simscape
  Scale : Subsystem
  Solver Configuration : nesl_utility/Solver Configuration  PhysicalDomain=network_engine_domain  SubClassName=solver  LeftPortType=input  RightPortType=generic  Tones=[]  Harmonics=[]  SimulateNoise=off  Profile=off  UseLocalSampling=off  EnableSwitchedLinearOptims=on  FrequencyDomain=off  UseCCode=off  RelTol=0.001  AbsTol=1e-06  MinStep=1e-09  ToWorkspace=off  RevertToSquareIcSolve=off  NumHomotopyIterations=100  PhasorMode=off  PhasorModeNumHarmonics=1  ConsistencySolver=NEWTON_FTOL  IndexReductionMethod=DerivativeReplacement  DoDC=off  ResidualTolerance=1e-09  ConsistencyTolSource=GLOBAL  ConsistencyAbsTol=0.001  ConsistencyRelTol=0.001  ConsistencyTolFactor=0.001  UseLocalSolver=on  LocalSolverChoice=NE_PARTITIONING_ADVANCER  ResolveIndetEquations=on  FunctionEvalNumThread=1  LocalSolverSampleTime=Ts_motor_simscape  DoFixedCost=on  MaxNonlinIter=4  MaxModeIter=2  ComputeImpulses=off  ImpulseIterations=1  LinearAlgebra=auto  LinearAlgebraNumThread=0  EquationFormulation=NE_TIME_EF  DelaysMemoryBudget=1024  AutomaticFiltering=on  FilteringTimeConstant=0.001  PartitionStorageMethod=AS_NEEDED  PartitionMemoryBudget=1024  PartitionMethod=ROBUST  MultibodyUseLocalSolver=off  MultibodyLocalSolverChoice=ODE1  MultibodyLocalSolverSampleTime=0.001
  Subsystem1 : Subsystem
  Terminator : Terminator
  measVI : Subsystem
  Iabc : Outport
  Hall : Outport  Port=2
  wires:
  Load/1 -> Rate Transition3/1
  Scale/1(ModWave) -> 6-pulse PWM generator/1(ModWave)
  Duty_Cycles/1 -> Rate Transition2/1
  Rate Transition3/1 -> Subsystem1/1(Tm)
  [Vabc] -> Terminator/1
  [HallSim] -> Hall/1  "Hall_Sensors"
  Rate Transition2/1 -> Scale/1(duty_abc)
  [Iabc] -> Iabc/1
  6-pulse PWM generator/1(g) -> 3phase converter/1(g)
  connections:
  Solver Configuration/RConn1 -- 3phase converter/RConn2 -- DC Voltage Source/RConn1 -- Electrical Reference1/LConn1
  BLDC Motor/LConn1 -- measVI/RConn1
  measVI/LConn1 -- 3phase converter/LConn1
  BLDC Motor/RConn2 -- Mechanical Rotational Reference/LConn1
  BLDC Motor/RConn1 -- Subsystem1/RConn1
  DC Voltage Source/LConn1 -- 3phase converter/RConn1

== system bldc_sixstep_f28069mLaunchPad/Inverter and Motor/Load_Profile (Torque) ==
  Data Type Conversion : DataTypeConversion  OutDataTypeStr=single  SaturateOnIntegerOverflow=off  RndMeth=Floor
  IIR Filter : mcbcontrolslib/IIR Filter  VariantControl=Low Pass Filter  VariantSelect=Low-pass  Filter_constant=0.01  advancedSettings=off  Ts=50e-6  cutOff_freq=32.1525
  "Motor Load reverse " : Constant  Value=-0.5*bldc.T_rated  OutDataTypeStr=dataType  SampleTime=-1
  Reversal : Step  Time=1.2  SampleTime=Ts_simulink
  Switch : Switch  Criteria=u2 > Threshold  SaturateOnIntegerOverflow=off  InputSameDT=off
  T_load : Step  Time=0.8  Before=0.05*bldc.T_rated  After=0.5*bldc.T_rated  SampleTime=Ts_simulink
  Load_Trq : Outport  VectorParamsAs1DForOutWhenUnconnected=off
  tag scope: Load_test=global
  wires:
  Data Type Conversion/1 -> IIR Filter/1
  IIR Filter/1 -> Load_Trq/1
  Switch/1 -> Data Type Conversion/1
  Reversal/1 -> Switch/2
  T_load/1 -> [Load_test], Switch/3  "Load"
  "Motor Load reverse "/1 -> Switch/1

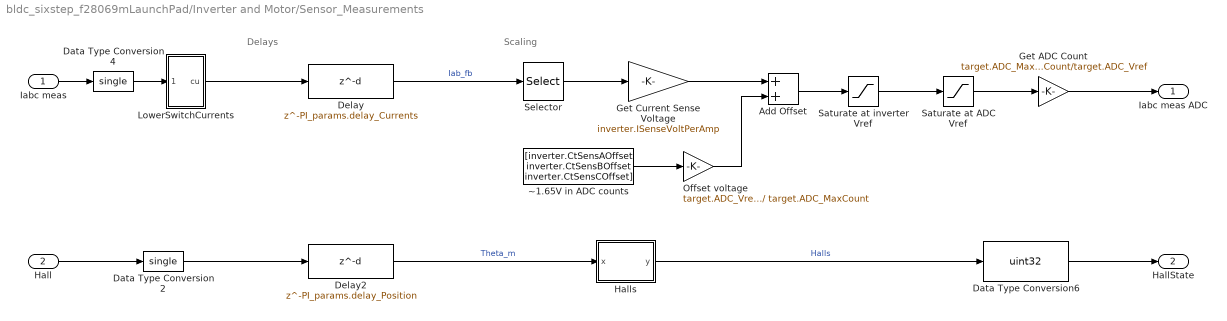
== system bldc_sixstep_f28069mLaunchPad/Inverter and Motor/Sensor_Measurements ==
  note: Scaling
  note: Delays
  Iabc meas : Inport
  Hall : Inport  Port=2
  Add Offset : Sum  RndMeth=Simplest
  Data Type Conversion2 : DataTypeConversion  OutDataTypeStr=single  RndMeth=Simplest  SaturateOnIntegerOverflow=off
  Data Type Conversion4 : DataTypeConversion  OutDataTypeStr=single  RndMeth=Simplest  SaturateOnIntegerOverflow=off
  Data Type Conversion6 : DataTypeConversion  OutDataTypeStr=uint32  SaturateOnIntegerOverflow=off  RndMeth=Floor
  Delay : Delay  DelayLength=PI_params.delay_Currents
  Delay2 : Delay  DelayLength=PI_params.delay_Position
  Get ADC Count : Gain  Gain=target.ADC_MaxCount/target.ADC_Vref  OutMin=0  OutMax=target.ADC_MaxCount  OutDataTypeStr=uint16  RndMeth=Simplest
  Get Current Sense Voltage : Gain  Gain=inverter.ISenseVoltPerAmp  RndMeth=Simplest  OutDataTypeStr=Inherit: Same as input
  Halls : Subsystem
  LowerSwitchCurrents : Subsystem
  Offset voltage : Gain  Gain=target.ADC_Vref / target.ADC_MaxCount  RndMeth=Simplest
  Saturate at ADC Vref : Saturate  UpperLimit=target.ADC_Vref  LowerLimit=0
  Saturate at inverter Vref : Saturate  UpperLimit=inverter.ISenseVref  LowerLimit=0
  Selector : Selector  InputPortWidth=3  IndexOptions=Index vector (dialog)  Indices=[1 2 3]  OutputSizes=1
  ~1.65V in ADC counts : Constant  Value="[inverter.CtSensAOffset inverter.CtSensBOffset  inverter.CtSensCOffset]"  OutDataTypeStr=single  SampleTime=-1
  Iabc meas ADC : Outport  VectorParamsAs1DForOutWhenUnconnected=off
  HallState : Outport  Port=2
  wires:
  Delay/1 -> Selector/1  "Iab_fb"
  Data Type Conversion4/1 -> LowerSwitchCurrents/1(In1)
  Iabc meas/1 -> Data Type Conversion4/1
  Hall/1 -> Data Type Conversion2/1
  Data Type Conversion2/1 -> Delay2/1
  Delay2/1 -> Halls/1(x)  "Theta_m"
  Halls/1(y) -> Data Type Conversion6/1  "Halls"
  Data Type Conversion6/1 -> HallState/1
  LowerSwitchCurrents/1(cu) -> Delay/1
  Saturate at inverter Vref/1 -> Saturate at ADC Vref/1
  Add Offset/1 -> Saturate at inverter Vref/1
  ~1.65V in ADC counts/1 -> Offset voltage/1
  Offset voltage/1 -> Add Offset/2
  Get Current Sense Voltage/1 -> Add Offset/1
  Get ADC Count/1 -> Iabc meas ADC/1
  Saturate at ADC Vref/1 -> Get ADC Count/1
  Selector/1 -> Get Current Sense Voltage/1

== system bldc_sixstep_f28069mLaunchPad/Serial receive/Data conditioning ==
  Rx_In : Inport
  Data Type Conversion1 : DataTypeConversion  OutDataTypeStr=single  RndMeth=Simplest  SaturateOnIntegerOverflow=off
  Data Type Conversion2 : DataTypeConversion  OutDataTypeStr=fixdt(1,16,12)  ConvertRealWorld=Stored Integer (SI)  RndMeth=Simplest  SaturateOnIntegerOverflow=off
  Rx_Out : Outport  VectorParamsAs1DForOutWhenUnconnected=off
  wires:
  Data Type Conversion1/1 -> Rx_Out/1
  Rx_In/1 -> Data Type Conversion2/1
  Data Type Conversion2/1 -> Data Type Conversion1/1

== system bldc_sixstep_f28069mLaunchPad/Serial receive/SCI_Rx ==
  Data Type Conversion : DataTypeConversion  OutDataTypeStr=fixdt(1,16,12)  RndMeth=Simplest  SaturateOnIntegerOverflow=off
  Data Type Conversion2 : DataTypeConversion  OutDataTypeStr=single  RndMeth=Simplest  SaturateOnIntegerOverflow=off
  Data Type Conversion3 : DataTypeConversion  OutDataTypeStr=uint16  ConvertRealWorld=Stored Integer (SI)  RndMeth=Simplest  SaturateOnIntegerOverflow=off
  Data Type Conversion4 : DataTypeConversion  OutDataTypeStr=single  RndMeth=Simplest  SaturateOnIntegerOverflow=off
  Enable : Constant  OutDataTypeStr=dataType  SampleTime=-1
  Mux : Mux  Inputs=2
  Reversal : Step  Time=1.2
  Speed_Ref_Final (rpm) : Constant  Value=-0.8*bldc.N_base  OutDataTypeStr=dataType  SampleTime=-1
  Speed_Ref_Init (rpm) : Step  Time=0.5  Before=0.2*bldc.N_base  After=0.8*bldc.N_base
  Switch : Switch  Criteria=u2 > Threshold  SaturateOnIntegerOverflow=off  InputSameDT=off
  rpm2PU : Gain  Gain=1/bldc.N_base  RndMeth=Simplest  OutDataTypeStr=Inherit: Same as input
  Data : Outport
  wires:
  Data Type Conversion2/1 -> Mux/1
  Speed_Ref_Init (rpm)/1 -> Switch/3
  Data Type Conversion3/1 -> Data/1
  Data Type Conversion/1 -> Data Type Conversion3/1
  rpm2PU/1 -> Data Type Conversion2/1
  Reversal/1 -> Switch/2
  Mux/1 -> Data Type Conversion/1
  Speed_Ref_Final (rpm)/1 -> Switch/1
  Enable/1 -> Data Type Conversion4/1
  Switch/1 -> rpm2PU/1
  Data Type Conversion4/1 -> Mux/2
